simulink model "asig_directa_final"  (R2020b)
settings: Solver=FixedStepDiscrete  StartTime=0.0  StopTime=Inf  FixedStep=0.001  RelTol=1e-3  EnableMultiTasking=on
values from neighbouring files (symbols this model uses):
  Gtd = c2d(Gt,T,'Tustin')    [demo.m]    (also in pendulo_modelo.m)
  Hd = place(Gtd.A',Gtd.C',pobsDiscrete)'    [demo.m]    (also in pendulo_modelo.m)
  Klqr = dlqr(Gtd.A,Gtd.B,Q,R)    [demo.m]    (also in pendulo_modelo.m)
  Robs = [1 0 ... (first row only)    [demo.m]    (also in pendulo_modelo.m)
  T = 0.001    [demo.m]    (also in pendulo_modelo.m)
undefined symbols (not defined in the file or in its folder): Discrete, Time
libraries: simulink x2, arduinolib x2, ctrlSharedLib x1
settings Model: SILPILModeSetting=veronly  ExtModeTrigDuration=2  Creator=aleca  LastModifiedBy=aleca
settings OptimizationCC: EnhancedBackFolding=on  PassReuseOutputArgsAs=Individual arguments  ZeroExternalMemoryAtStartup=off  ZeroInternalMemoryAtStartup=off  MaxStackSize=64  OptimizeBlockOrder=speed  DifferentSizesBufferReuse=on  OptimizationCustomize=off  EfficientTunableParamExpr=on
settings DebuggingCC: ParameterTunabilityLossMsg=error
settings HardwareCC: ProdBitPerInt=16  ProdBitPerPointer=16  ProdBitPerSizeT=16  ProdBitPerPtrDiffT=16  ProdLargestAtomicFloat=None  ProdWordSize=8  ProdHWDeviceType=Atmel->AVR  UseEmbeddedCoderFeatures=off  UseSimulinkCoderFeatures=off
settings SFSimCC: MATLABDynamicMemAlloc=off
settings RTWCC: Description=Embedded Coder  SystemTargetFile=ert.tlc  HardwareBoard=Arduino Mega 2560  TemplateMakefile=ert_default_tmf  Toolchain=Arduino AVR  BuildConfiguration=Faster Runs
settings CodeAppCC: ForceParamTrailComments=on  IgnoreCustomStorageClasses=off  OperatorAnnotations=on  SimulinkDataObjDesc=on  SFDataObjDesc=on  InsertBlockDesc=on
settings ERTTargetCC: SupportContinuousTime=on  SupportNonInlinedSFcns=on  SupportVariableSizeSignals=on  ExtModeStaticAllocSize=2048

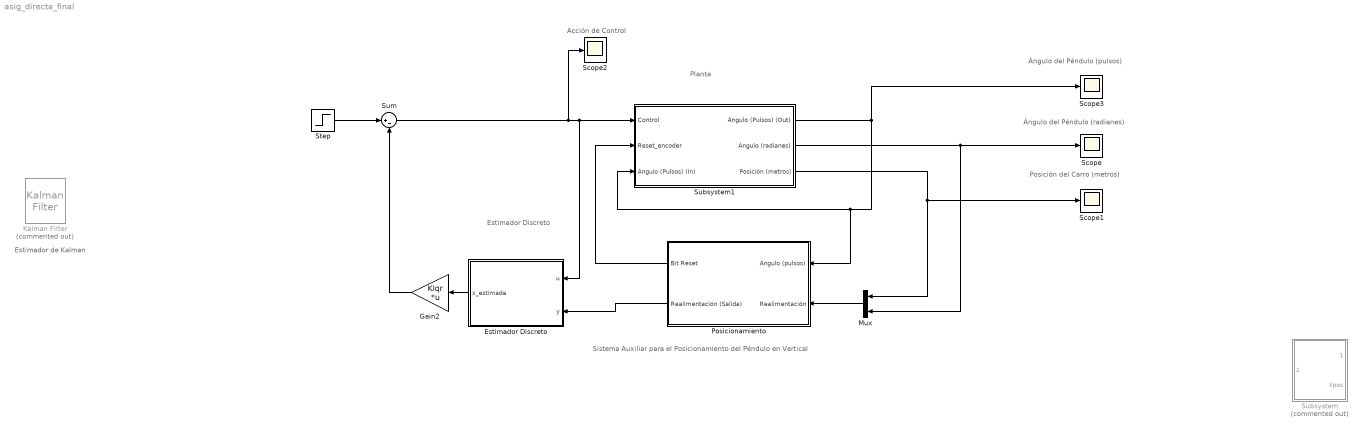
== system asig_directa_final ==
  note: Planta
  note: Acción de Control
  note: Estimador
      | Discreto
  note: Posición del Carro (metros)
  note: Ángulo del Péndulo (radianes)
  note: Sistema Auxiliar para el Posicionamiento del Péndulo en Vertical
  note: Ángulo del Péndulo (pulsos)
  note: Estimador
      | de Kalman
  Estimador Discreto : Subsystem
      settings: PortSchema="{\"entries\":[{\"content\":{\"sides\":[{\"content\":{\"connectorIds\":[\"Out1\"]},\"type\":\"ConnectorPlacement.EquallySpacedRectSide\",\"uuid\":\"54c951a6-c492-466a-87cc-2666df80341c\"},{\"content\":{\"connectorIds\":[\"In1\",\"In2\"],\"side\":\"RIGHT\"},\"type\":\"ConnectorPlacement.EquallySpacedRectSide\",\"uuid\":\"84d159db-5f82-478e-80b7-0aa3e5947a31\"},{\"content\":{\"connectorIds\":[],\"side\":\"TOP\"},\"type\":\"ConnectorPlacement.EquallySpacedRectSide\",\"uuid\":\"30ac016a-f884-45ce-a1da-2e3ef49bb594\"},{\"content\":{\"connectorIds\":[],\"side\":\"HIDDEN\"},\"type\":\"ConnectorPlacement.EquallySpacedRectSide\",\"uuid\":\"fc69af6f-3ea5-4985-ad9c-b3efd3bcb5d5\"}]},\"type\":\"ConnectorPlacement.EquallySpacedConnector\",\"uuid\":\"efc1973c-7238-45a0-b3a7-e4369d7e03c8\"}],\"packageUris\":[\"http://schema.mathworks.com/mf0/Connector/R2020b\"],\"version\":\"1.0\"}"
  Gain2 : Gain  Gain=Klqr  Multiplication=Matrix(K*u)
  Kalman Filter : ctrlSharedLib/Kalman Filter  Commented=on  TimeDomain=Discrete-Time  UseCurrentEstimator=off  ModelSource=Individual A, B, C, D matrices  ModelSourceVariable=ss(0.95,1,1,0,1)  A=Gtd.A  B=Gtd.B  C=Gtd.C  D=Gtd.D  NumberOfStates=1  NumberOfInputs=1  NumberOfOutputs=1  InitialEstimateSource=Dialog  X0=0  P0=10  UseK=off  UseGH=off  NumberOfProcessNoiseInputs=1  G=1  TimeInvariantG=on  H=0  TimeInvariantH=on  Q=Qobs  TimeInvariantQ=on  R=Robs  TimeInvariantR=on  N=0  TimeInvariantN=on  AddInputPort=on  AddEnablePort=off  OutputEstimatedY=off  OutputP=off  Ts=-1
  Mux : Mux  Inputs=2
  Posicionamiento : Subsystem
  Scope{,1..3} (4 alike) : Scope
  Step : Step  After=0  SampleTime=0.001
  Subsystem : Subsystem  Commented=on
  Subsystem1 : Subsystem
  Sum : Sum  Inputs=|+-
  wires:
  Step/1 -> Sum/1
  Gain2/1 -> Sum/2
  Mux/1 -> Posicionamiento/2(Realimentación)
  Sum/1 -> Estimador Discreto/1(u), Subsystem1/1(Control), Scope2/1
  Subsystem1/3(Posición (metros)) -> Mux/1, Scope1/1
  Subsystem1/1(Ángulo (Pulsos) (Out)) -> Subsystem1/3(Ángulo (Pulsos) (In)), Posicionamiento/1(Ángulo (pulsos)), Scope3/1
  Subsystem1/2(Ángulo (radianes)) -> Mux/2, Scope/1
  Posicionamiento/1(Bit Reset) -> Subsystem1/2(Reset_encoder)
  Posicionamiento/2(Realimentación (Salida)) -> Estimador Discreto/2(y)
  Estimador Discreto/1(x_estimada) -> Gain2/1

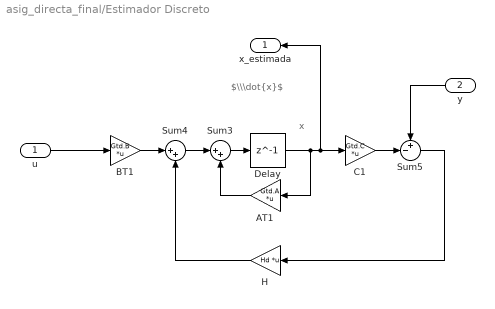
== system asig_directa_final/Estimador Discreto ==
  note: $\\\dot{x}$
  note: x
  u : Inport
  y : Inport  Port=2
  AT1 : Gain  Gain=Gtd.A  Multiplication=Matrix(K*u)
  BT1 : Gain  Gain=Gtd.B  Multiplication=Matrix(K*u)
  C1 : Gain  Gain=Gtd.C  Multiplication=Matrix(K*u)
  Delay : Delay  DelayLength=1
  H : Gain  Gain=Hd  Multiplication=Matrix(K*u)
  Sum3 : Sum  Inputs=|++
  Sum4 : Sum  Inputs=|++
  Sum5 : Sum  Inputs=+-|
  x_estimada : Outport
  wires:
  BT1/1 -> Sum4/1
  Delay/1 -> x_estimada/1, C1/1, AT1/1
  Sum3/1 -> Delay/1
  y/1 -> Sum5/1
  Sum4/1 -> Sum3/1
  H/1 -> Sum4/2
  C1/1 -> Sum5/2
  AT1/1 -> Sum3/2
  Sum5/1 -> H/1
  u/1 -> BT1/1

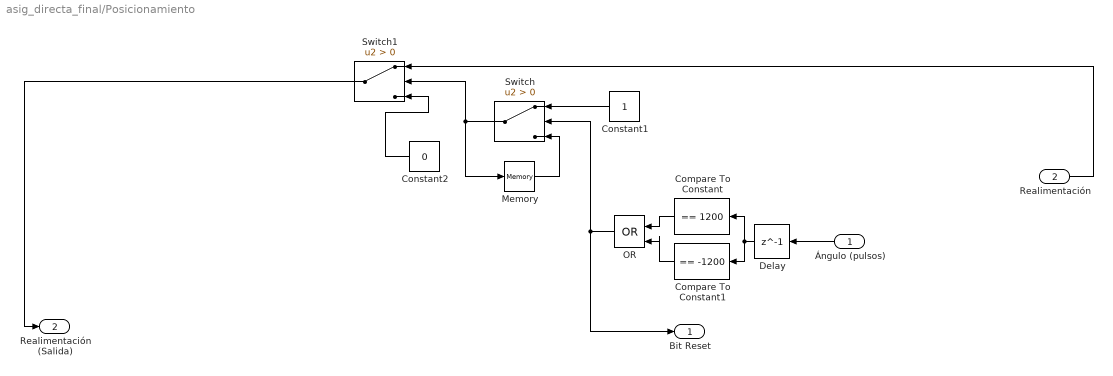
== system asig_directa_final/Posicionamiento ==
  Ángulo (pulsos) : Inport
  Realimentación : Inport  Port=2
  Compare To Constant : simulink/Logic and Bit Operations/Compare To Constant  relop===  const=1200  OutDataTypeStr=boolean
  Compare To Constant1 : simulink/Logic and Bit Operations/Compare To Constant  relop===  const=-1200  OutDataTypeStr=boolean
  Constant1 : Constant  OutDataTypeStr=boolean  SampleTime=-1
  Constant2 : Constant  Value=0  SampleTime=-1
  Delay : Delay  DelayLength=1
  Memory : Memory  InheritSampleTime=on
  OR : Logic  Operator=OR  IconShape=distinctive  AllPortsSameDT=off  OutDataTypeStr=boolean
  Switch : Switch  Criteria=u2 > Threshold
  Switch1 : Switch  Criteria=u2 > Threshold
  Bit Reset : Outport
  Realimentación (Salida) : Outport  Port=2
  wires:
  Memory/1 -> Switch/3
  Switch/1 -> Switch1/2, Memory/1
  Compare To Constant1/1 -> OR/2
  Compare To Constant/1 -> OR/1
  Delay/1 -> Compare To Constant/1, Compare To Constant1/1
  Constant2/1 -> Switch1/3
  OR/1 -> Bit Reset/1, Switch/2
  Realimentación/1 -> Switch1/1
  Constant1/1 -> Switch/1
  Switch1/1 -> Realimentación (Salida)/1
  Ángulo (pulsos)/1 -> Delay/1

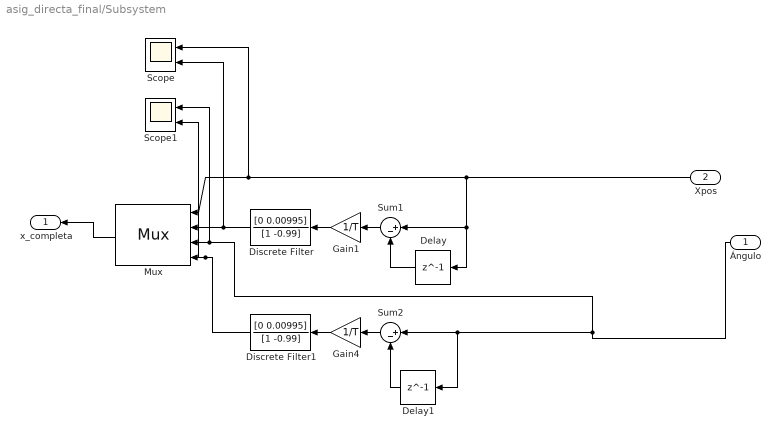
== system asig_directa_final/Subsystem ==
  Ángulo : Inport
  Xpos : Inport  Port=2
  Delay : Delay  DelayLength=1
  Delay1 : Delay  DelayLength=1
  Discrete Filter : DiscreteFilter  Numerator=[0 0.00995]  Denominator=[1 -0.99]
  Discrete Filter1 : DiscreteFilter  Numerator=[0 0.00995]  Denominator=[1 -0.99]
  Gain1 : Gain  Gain=1/T
  Gain4 : Gain  Gain=1/T
  Mux : Mux
      settings: DisplayOption=signals
  Scope : Scope  NumInputPorts=2
  Scope1 : Scope  NumInputPorts=2
  Sum1 : Sum  Inputs=|+-
  Sum2 : Sum  Inputs=|+-
  x_completa : Outport
  wires:
  Ángulo/1 -> Scope1/1, Mux/3, Sum2/1, Delay1/1
  Delay1/1 -> Sum2/2
  Gain4/1 -> Discrete Filter1/1
  Xpos/1 -> Delay/1, Sum1/1, Scope/1, Mux/1
  Sum2/1 -> Gain4/1
  Gain1/1 -> Discrete Filter/1
  Sum1/1 -> Gain1/1
  Delay/1 -> Sum1/2
  Mux/1 -> x_completa/1
  Discrete Filter/1 -> Scope/2, Mux/2
  Discrete Filter1/1 -> Scope1/2, Mux/4

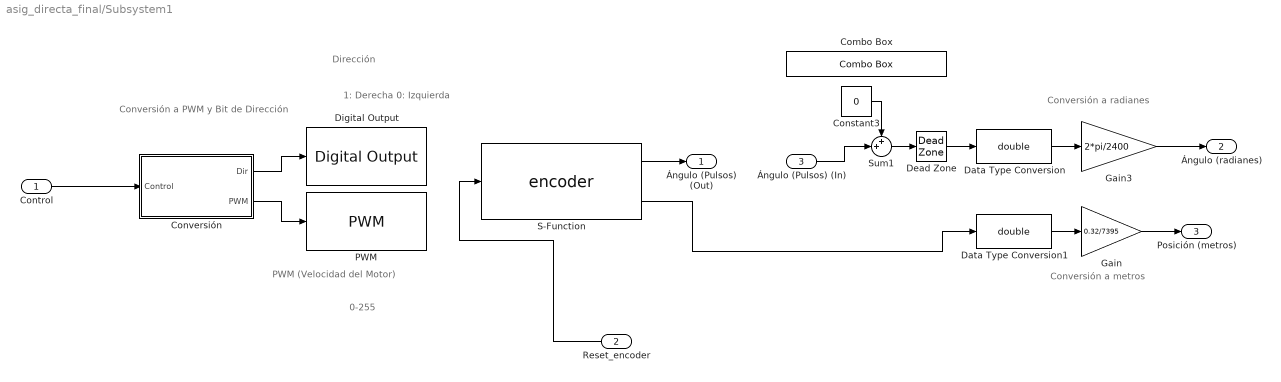
== system asig_directa_final/Subsystem1 ==
  note: Conversión a metros
  note: Dirección
  note: PWM (Velocidad del Motor)
  note: 1: Derecha
      | 0: Izquierda
  note: Conversión a radianes
  note: 0-255
  note: Conversión a PWM y
      | Bit de Dirección
  Control : Inport
  Reset_encoder : Inport  Port=2
  Ángulo (Pulsos) (In) : Inport  Port=3
  Combo Box : ComboBox  LabelPosition=Hide  SelectedLabel=0
      settings: Values={{'0', '1', '2', '-2', '-1'}, [0 1 2 -2 -1]}
  Constant3 : Constant  Value=0  SampleTime=-1
  Conversión : Subsystem
  Data Type Conversion : DataTypeConversion  OutDataTypeStr=double
  Data Type Conversion1 : DataTypeConversion  OutDataTypeStr=double
  Dead Zone : DeadZone  LowerValue=0  UpperValue=0  SaturateOnIntegerOverflow=on
  Digital Output : arduinolib/Digital Output  pinNumber=10  Direction=output  blockPlatform=arduino
  Gain : Gain  Gain=0.32/7395
  Gain3 : Gain  Gain=2*pi/2400
  PWM : arduinolib/PWM  pinNumber=9  frequencyType=Default  desiredFrequency=490.2  achievableFrequency=490.2
  S-Function : S-Function  FunctionName=encoder  SFunctionModules='encoder_wrapper'  SFunctionDeploymentMode=off  EnableBusSupport=off
  Sum1 : Sum  Inputs=++|
  Ángulo (Pulsos) (Out) : Outport
  Ángulo (radianes) : Outport  Port=2
  Posición (metros) : Outport  Port=3
  wires:
  Gain/1 -> Posición (metros)/1
  Sum1/1 -> Dead Zone/1
  Conversión/1(Dir) -> Digital Output/1
  Conversión/2(PWM) -> PWM/1
  Dead Zone/1 -> Data Type Conversion/1
  Data Type Conversion/1 -> Gain3/1
  Constant3/1 -> Sum1/1
  S-Function/2 -> Data Type Conversion1/1
  Data Type Conversion1/1 -> Gain/1
  S-Function/1 -> Ángulo (Pulsos) (Out)/1
  Reset_encoder/1 -> S-Function/1
  Control/1 -> Conversión/1(Control)
  Gain3/1 -> Ángulo (radianes)/1
  Ángulo (Pulsos) (In)/1 -> Sum1/2

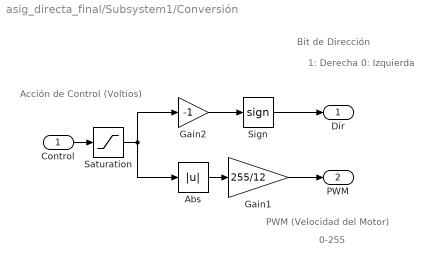
== system asig_directa_final/Subsystem1/Conversión ==
  note: Acción de Control
      | (Voltios)
  note: Bit de Dirección
  note: 1: Derecha
      | 0: Izquierda
  note: 0-255
  note: PWM (Velocidad del Motor)
  Control : Inport
  Abs : Abs
  Gain1 : Gain  Gain=255/12
  Gain2 : Gain  Gain=-1
  Saturation : Saturate  UpperLimit=12  LowerLimit=-12
  Sign : Signum
  Dir : Outport
  PWM : Outport  Port=2
  wires:
  Abs/1 -> Gain1/1
  Gain1/1 -> PWM/1
  Control/1 -> Saturation/1
  Saturation/1 -> Gain2/1, Abs/1
  Sign/1 -> Dir/1
  Gain2/1 -> Sign/1
